simulink model "point_4_2_3"  (Simulink 7.5)
settings: Solver=ode45  StartTime=0.0  StopTime=3.0  RelTol=1e-3
settings Model: Creator=davito  LastModifiedBy=davito

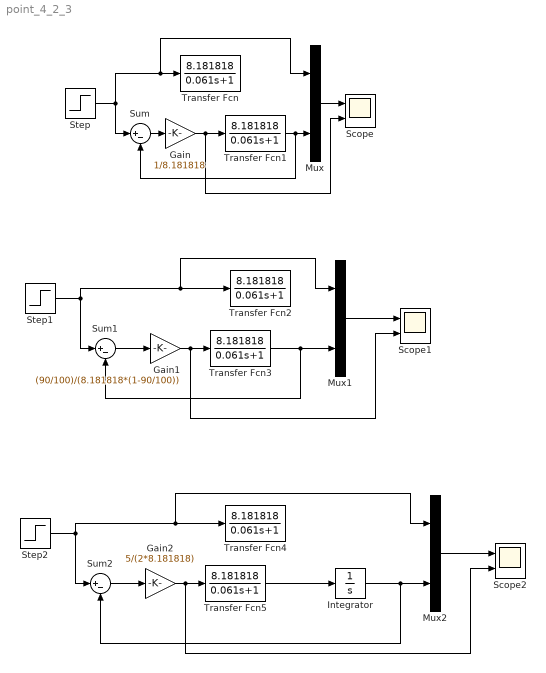
== system point_4_2_3 ==
  Gain : Gain  Gain=1/8.181818  ParameterDataType=fixdt(1, 16)  ParameterScaling=2^0  OutDataType=fixdt(1, 16)  OutScaling=2^0
  Gain1 : Gain  Gain=(90/100)/(8.181818*(1-90/100))  ParameterDataType=fixdt(1, 16)  ParameterScaling=2^0  OutDataType=fixdt(1, 16)  OutScaling=2^0
  Gain2 : Gain  Gain=5/(2*8.181818)  ParameterDataType=fixdt(1, 16)  ParameterScaling=2^0  OutDataType=fixdt(1, 16)  OutScaling=2^0
  Integrator : Integrator
  Mux : Mux  Inputs=2
  Mux1 : Mux  Inputs=2
  Mux2 : Mux  Inputs=2
  Scope : Scope  NumInputPorts=2
      settings: YMin=-5~-5  YMax=5~5
  Scope1 : Scope  NumInputPorts=2
      settings: YMin=-5~-5  YMax=5~5
  Scope2 : Scope  NumInputPorts=2
      settings: YMin=0~-1  YMax=110~32  SaveName=ScopeData2
  Step : Step  Time=0  After=100  SampleTime=0
  Step1 : Step  Time=0  After=100  SampleTime=0
  Step2 : Step  Time=0  After=100  SampleTime=0
  Sum : Sum  Inputs=|+-  OutDataType=fixdt(1, 16)  OutScaling=2^0
  Sum1 : Sum  Inputs=|+-  OutDataType=fixdt(1, 16)  OutScaling=2^0
  Sum2 : Sum  Inputs=|+-  OutDataType=fixdt(1, 16)  OutScaling=2^0
  Transfer Fcn{,1..5} (6 alike) : TransferFcn  Numerator=[8.181818]  Denominator=[0.061 1]
  wires:
  Step/1 -> Transfer Fcn/1, Mux/1, Sum/1
  Mux/1 -> Scope/1
  Sum/1 -> Gain/1
  Transfer Fcn1/1 -> Mux/2, Sum/2
  Gain/1 -> Transfer Fcn1/1, Scope/2
  Step1/1 -> Sum1/1, Transfer Fcn2/1, Mux1/1
  Mux1/1 -> Scope1/1
  Sum1/1 -> Gain1/1
  Transfer Fcn3/1 -> Sum1/2, Mux1/2
  Gain1/1 -> Transfer Fcn3/1, Scope1/2
  Step2/1 -> Transfer Fcn4/1, Mux2/1, Sum2/1
  Mux2/1 -> Scope2/1
  Sum2/1 -> Gain2/1
  Transfer Fcn5/1 -> Integrator/1
  Gain2/1 -> Transfer Fcn5/1, Scope2/2
  Integrator/1 -> Mux2/2, Sum2/2
